simulink model "Deepa_ibvsCt1"  (R2016b)
settings: Solver=ode45  StartTime=0.0  StopTime=5  RelTol=1e-3  EnableMultiTasking=on
InitFcn:
  | cam = CentralCamera('default')
undefined symbols (not defined in the file): mkgrid, p560, transl, trotz
libraries: roblocks x14
settings Model: ExtModeTrigMode=oneshot  ExtModeArmWhenConnect=off  Creator=pic  LastModifiedBy=deela
settings DataIOCC: SaveFormat=Structure  SignalLoggingSaveFormat=ModelDataLogs  ReturnWorkspaceOutputs=on
settings OptimizationCC: BlockReduction=off  BooleanDataType=off  ExpressionDepthLimit=2147483647  InitFltsAndDblsToZero=on  LifeSpan=inf
settings DebuggingCC: SaveWithParameterizedLinksMsg=none  UnderspecifiedInitializationDetection=Classic  MergeDetectMultiDrivingBlocksExec=none  SignalResolutionControl=TryResolveAllWithWarning  MultiTaskDSMMsg=warning  MultiTaskCondExecSysMsg=none  FcnCallInpInsideContextMsg=warning  StateNameClashWarn=warning  SFUnexpectedBacktrackingDiag=warning  SFNoUnconditionalDefaultTransitionDiag=warning  SFExecutionAtInitializationDiag=none
settings HardwareCC: ProdBitPerPointer=32  ProdBitPerSizeT=32  ProdBitPerPtrDiffT=32  ProdLargestAtomicFloat=None  ProdIntDivRoundTo=Undefined  ProdEndianess=Unspecified  ProdWordSize=32  ProdHWDeviceType=32-bit Generic  TargetUnknown=on
settings ModelReferenceCC: PropagateSignalLabelsOutOfModel=off
settings GRTTargetCC: TargetLangStandard=C89/C90 (ANSI)  ModelReferenceCompliant=off  CompOptLevelCompliant=off  GeneratePreprocessorConditionals=Disable all  CombineOutputUpdateFcns=off  MatFileLogging=off  GRTInterface=on
settings ConfigComp: CovMetricSettings=dw  CovHtmlReporting=on  CovSaveCumulativeToWorkspaceVar=on  CovSaveSingleToWorkspaceVar=on  CovExternalEMLEnable=off

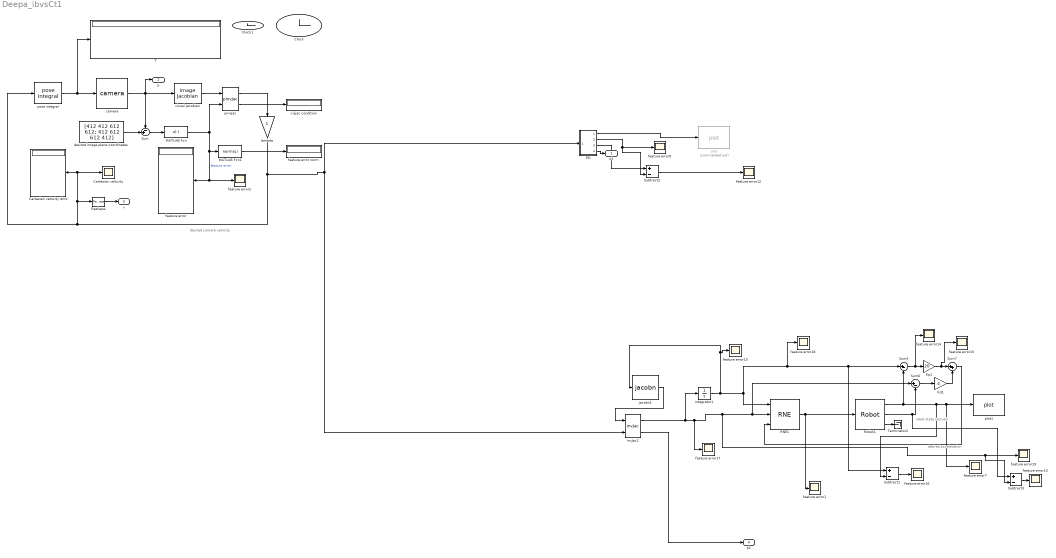
== system Deepa_ibvsCt1 ==
  note: desired camera velocity
  note: robot state
      | (actual)
  note: desired acceleration
  Cartesian velocity : Scope
  Cartesian velocity dmd : Display
      settings: Format=bank
  Clock : Clock
  Clock1 : Clock
  Integrator1 : Integrator
  Kd1 : Gain  Gain=4  SaturateOnIntegerOverflow=on  OutDataTypeStr=Inherit: Same as input  ParamDataTypeStr=Inherit: Same as input
  Kp1 : Gain  Gain=20  SaturateOnIntegerOverflow=on  OutDataTypeStr=Inherit: Same as input  ParamDataTypeStr=Inherit: Same as input
  MATLAB Fcn : MATLABFcn  MATLABFcn=u(:)  Output1D=off
  MATLAB Fcn1 : MATLABFcn  MATLABFcn=norm(u)
  PD : Subsystem
  RNE1 : roblocks/Dynamics/RNE  robot=p560.nofriction()  grav=[0 0 9.81]
  Reshape : Reshape  OutputDimensionality=Customize  OutputDimensions=6
  Robot1 : roblocks/Dynamics/Robot  robot=p560.nofriction()  q0=[0 0 0 0 0 0]
  Subtract1 : Sum  Inputs=+-
  Subtract2 : Sum  Inputs=+-
  Subtract3 : Sum  Inputs=+-
  Sum : Sum  Inputs=-+|  SaturateOnIntegerOverflow=on  InputSameDT=on  OutDataTypeStr=Inherit: Same as first input
  Sum5 : Sum  Inputs=|+-  SaturateOnIntegerOverflow=on  InputSameDT=on  OutDataTypeStr=Inherit: Same as first input
  Sum6 : Sum  Inputs=|+-  SaturateOnIntegerOverflow=on  InputSameDT=on  OutDataTypeStr=Inherit: Same as first input
  Sum7 : Sum  Inputs=|++  SaturateOnIntegerOverflow=on  InputSameDT=on  OutDataTypeStr=Inherit: Same as first input
  T : Display
  Terminator2 : Terminator
  camera : roblocks/Vision/camera  cam=cam  points=mkgrid(2, 0.5, transl(0,0,3))
  desired image plane coordinates : Constant  Value=[412 412 612 612; 412 612 612 412]  VectorParams1D=off
  feature error : Display
      settings: Format=bank
  feature error norm : Display
  feature error{1..2,7,9..10,12..19} (13 alike) : Scope
  invJac2 : roblocks/Vision/invJac
  jacobn1 : roblocks/Kinematics/jacobn  robot=p560
      link override MATLAB Fcn: MATLABFcn=jacobn(robot,u)
  lambda : Gain  SaturateOnIntegerOverflow=on  OutDataTypeStr=Inherit: Same as input  ParamDataTypeStr=Inherit: Same as input
  pinvJac : roblocks/Vision/pinvJac
  plot : roblocks/Robot Graphics/plot  Commented=on  robot=p560  fps=25  holdplot=on
  plot1 : roblocks/Robot Graphics/plot  robot=p560  fps=25  holdplot=on
  pose integral : roblocks/Kinematics/pose integral  T0=transl(0,0,1)*trotz(1.5)  dt=0.02
  visjac condition : Display
  visual Jacobian : roblocks/Vision/image Jacobian  cam=cam  z=3
  p1 : Outport
  p : Outport  Port=2
  v : Outport  Port=3
  p2 : Outport  Port=4
  wires:
  Subtract2/1 -> feature error12/1
  camera/1 -> Sum/1, visual Jacobian/1, p/1
  Sum/1 -> MATLAB Fcn/1
  desired image plane coordinates/1 -> Sum/2
  MATLAB Fcn/1 -> MATLAB Fcn1/1, feature error2/1, feature error/1, pinvJac/2  "feature error"
  pinvJac/2 -> visjac condition/1
  MATLAB Fcn1/1 -> feature error norm/1
  pinvJac/1 -> lambda/1
  pose integral/1 -> T/1, camera/1
  visual Jacobian/1 -> pinvJac/1
  Reshape/1 -> v/1
  Sum5/1 -> feature error14/1, Kp1/1
  Kp1/1 -> feature error15/1, Sum7/1
  Robot1/1 -> Sum5/2, Subtract1/2, feature error7/1, plot1/1
  Robot1/2 -> Subtract3/1, Sum6/2
  Sum6/1 -> Kd1/1
  Kd1/1 -> Sum7/2
  Robot1/3 -> Terminator2/1
  Sum7/1 -> RNE1/3
  RNE1/1 -> Robot1/1, feature error1/1
  Subtract1/1 -> feature error16/1
  Subtract3/1 -> feature error13/1
  invJac2/1 -> Subtract3/2, feature error19/1, Sum6/1, RNE1/2, feature error17/1, Integrator1/1
  jacobn1/1 -> invJac2/1
  invJac2/2 -> p2/1
  Integrator1/1 -> feature error10/1, jacobn1/1, RNE1/1, feature error18/1, Subtract1/1, Sum5/1
  lambda/1 -> PD/1(In1), invJac2/2, Cartesian velocity dmd/1, Cartesian velocity/1, Reshape/1, pose integral/1
  PD/2(Out2) -> Subtract2/2, feature error9/1
  PD/1(Out1) -> plot/1
  PD/3(Out3) -> Subtract2/1
  PD/4(Out4) -> p1/1

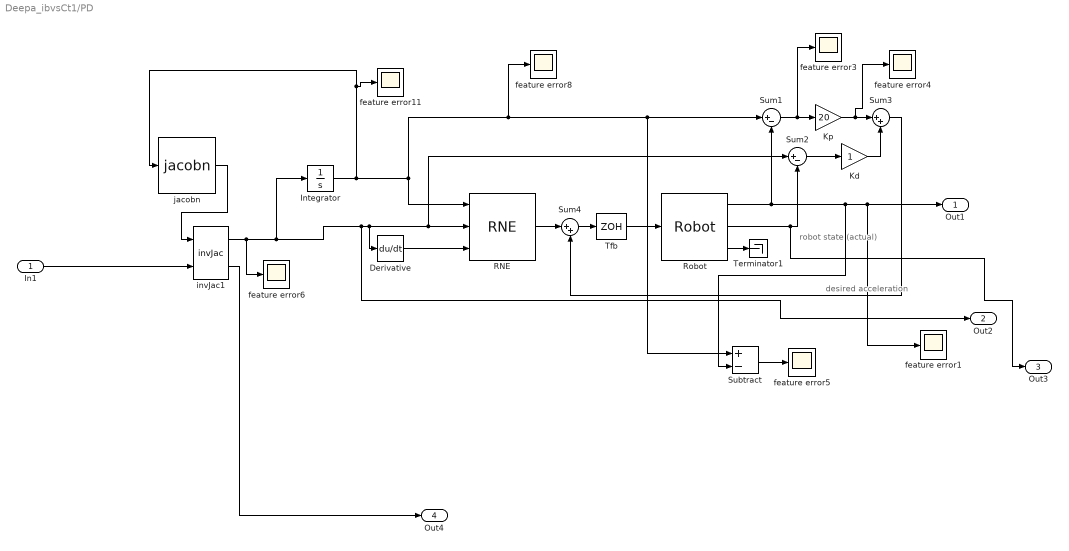
== system Deepa_ibvsCt1/PD ==
  note: robot state
      | (actual)
  note: desired acceleration
  In1 : Inport
  Derivative : Derivative
  Integrator : Integrator
  Kd : Gain  SaturateOnIntegerOverflow=on  OutDataTypeStr=Inherit: Same as input  ParamDataTypeStr=Inherit: Same as input
  Kp : Gain  Gain=20  SaturateOnIntegerOverflow=on  OutDataTypeStr=Inherit: Same as input  ParamDataTypeStr=Inherit: Same as input
  RNE : roblocks/Dynamics/RNE  robot=p560.nofriction()  grav=[0 0 9.81]
  Robot : roblocks/Dynamics/Robot  robot=p560.nofriction()  q0=[0 0 0 0 0 0]
  Subtract : Sum  Inputs=+-
  Sum1 : Sum  Inputs=|+-  SaturateOnIntegerOverflow=on  InputSameDT=on  OutDataTypeStr=Inherit: Same as first input
  Sum2 : Sum  Inputs=|+-  SaturateOnIntegerOverflow=on  InputSameDT=on  OutDataTypeStr=Inherit: Same as first input
  Sum3 : Sum  Inputs=|++  SaturateOnIntegerOverflow=on  InputSameDT=on  OutDataTypeStr=Inherit: Same as first input
  Sum4 : Sum  Inputs=|++
  Terminator1 : Terminator
  Tfb : ZeroOrderHold  SampleTime=0.01
  feature error{1,3..6,8,11} (7 alike) : Scope
  invJac1 : roblocks/Vision/invJac
  jacobn : roblocks/Kinematics/jacobn  robot=p560
      link override MATLAB Fcn: MATLABFcn=jacobn(robot,u)
  Out1 : Outport
  Out2 : Outport  Port=2
  Out3 : Outport  Port=3
  Out4 : Outport  Port=4
  wires:
  In1/1 -> invJac1/2
  Sum4/1 -> Tfb/1
  invJac1/1 -> feature error6/1, Integrator/1, Out2/1, Derivative/1, Sum2/1, RNE/2
  Integrator/1 -> feature error11/1, jacobn/1, RNE/1, feature error8/1, Subtract/1, Sum1/1
  invJac1/2 -> Out4/1
  Subtract/1 -> feature error5/1
  jacobn/1 -> invJac1/1
  Tfb/1 -> Robot/1
  Sum1/1 -> feature error3/1, Kp/1
  Robot/1 -> Sum1/2, Subtract/2, Out1/1, feature error1/1
  Kp/1 -> feature error4/1, Sum3/1
  Robot/2 -> Out3/1, Sum2/2
  Robot/3 -> Terminator1/1
  Sum3/1 -> Sum4/2
  RNE/1 -> Sum4/1
  Kd/1 -> Sum3/2
  Sum2/1 -> Kd/1
  Derivative/1 -> RNE/3
